simulink model "Design_Module_1"  (R2023b)
settings: Solver=VariableStepAuto  StartTime=0.0  StopTime=10  RelTol=1e-3
libraries: eeGeneralControl x2, dspsigops x1
settings Model: Creator=Tristan Ruel  LastModifiedBy=Tristan Ruel

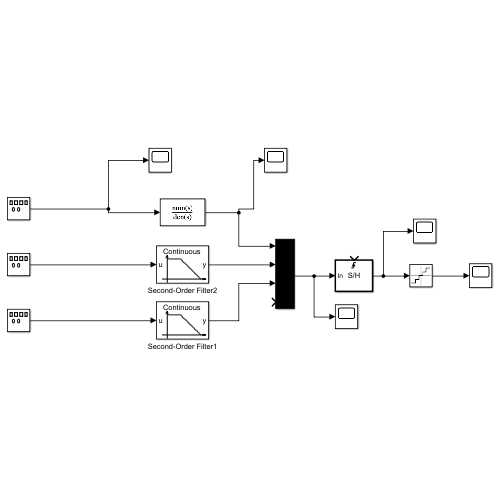
[thumbnail: Simulink's stored preview of the top-level diagram]
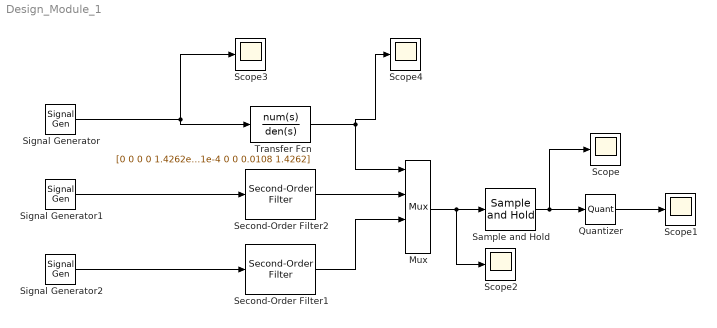
== system Design_Module_1 ==
  Mux : Mux
  Quantizer : Quantizer
  Sample and Hold : dspsigops/Sample and Hold  trig=Rising edge  initCond=0  latchinput=off
  Scope{,1..4} (5 alike) : Scope
  Second-Order Filter1 : eeGeneralControl/Second-Order Filter  FilterType=Low-pass  fn=60  Zeta=0.707  Ts=0  A0=0  Ph0=0  f0=0  b0=0
      settings: LibrarySourceBlock=ee_sl_lib/General Control/Second-Order Filter
  Second-Order Filter2 : eeGeneralControl/Second-Order Filter  FilterType=Low-pass  fn=60  Zeta=0.707  Ts=0  A0=0  Ph0=0  f0=0  b0=0
      settings: LibrarySourceBlock=ee_sl_lib/General Control/Second-Order Filter
  Signal Generator : SignalGenerator  Frequency=15
  Signal Generator1 : SignalGenerator  Amplitude=5  Frequency=20
  Signal Generator2 : SignalGenerator  Amplitude=5  Frequency=20
  Transfer Fcn : TransferFcn  Numerator=[0 0 0 0 1.4262e10]  Denominator=[1e-4 0 0 0.0108 1.4262]
  wires:
  Signal Generator2/1 -> Second-Order Filter1/1
  Signal Generator1/1 -> Second-Order Filter2/1
  Signal Generator/1 -> Transfer Fcn/1, Scope3/1
  Second-Order Filter1/1 -> Mux/3
  Second-Order Filter2/1 -> Mux/2
  Transfer Fcn/1 -> Scope4/1, Mux/1
  Sample and Hold/1 -> Scope/1, Quantizer/1
  Mux/1 -> Scope2/1, Sample and Hold/1
  Quantizer/1 -> Scope1/1
